simulink model "Seminar6_topic2"  (R2015b)
settings: Solver=VariableStepAuto  StartTime=0.0  StopTime=0.2  FixedStep=5e-8  MaxStep=1e-5  RelTol=1e-3  AbsTol=.01
libraries: powerlib x11, powerlib_meascontrol x1, simulink x1
settings Model: Creator=96547  LastModifiedBy=96547
settings DataIOCC: SaveFormat=Array  SignalLoggingSaveFormat=ModelDataLogs
settings OptimizationCC: InitFltsAndDblsToZero=on
settings DebuggingCC: SaveWithParameterizedLinksMsg=none  UnderspecifiedInitializationDetection=Classic  MergeDetectMultiDrivingBlocksExec=none  SignalResolutionControl=TryResolveAllWithWarning  SolverPrmCheckMsg=warning  MultiTaskDSMMsg=warning  MultiTaskCondExecSysMsg=none  FcnCallInpInsideContextMsg=EnableAllAsWarning  UnconnectedInputMsg=none  UnconnectedOutputMsg=none  UnconnectedLineMsg=none  AllowSymbolicDim=on
settings HardwareCC: ProdBitPerPointer=32  ProdLargestAtomicFloat=None  ProdIntDivRoundTo=Undefined  ProdEndianess=Unspecified  ProdWordSize=32  ProdHWDeviceType=32-bit Generic
settings SFSimCC: SimUseLocalCustomCode=on
settings RTWCC: RTWUseLocalCustomCode=on
settings GRTTargetCC: TargetFcnLib=ansi_tfl_tmw.mat  CombineOutputUpdateFcns=off  GRTInterface=on
settings ConfigComp: CovModelRefEnable=Off  CovExternalEMLEnable=on

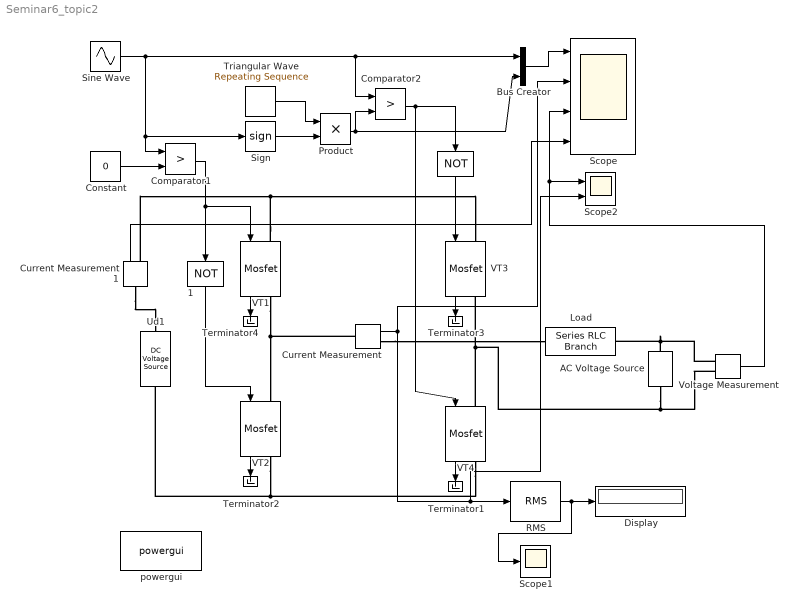
== system Seminar6_topic2 ==
  " " : Logic  Operator=NOT  AllPortsSameDT=off  OutDataTypeStr=boolean
  " 1" : Logic  Operator=NOT  AllPortsSameDT=off  OutDataTypeStr=boolean
  AC Voltage Source : powerlib/Electrical Sources/AC Voltage Source  Amplitude=220*sqrt(2)  Phase=0  Frequency=50  SampleTime=0  Measurements=None  BusType=swing  Pref=10e3  Qref=0  Qmin=-inf  Qmax=+inf
  Bus Creator : BusCreator  DialogController=Simulink.DDGSource_Bus  Inputs=2
  Comparator1 : RelationalOperator  Operator=>  OutDataTypeStr=boolean  ZeroCross=off
  Comparator2 : RelationalOperator  Operator=>  OutDataTypeStr=boolean  ZeroCross=off
  Constant : Constant  Value=0
  Current Measurement : powerlib/Measurements/Current Measurement  PhasorSimulation=off  OutputType=Complex  PSBequivalent=0
  Current Measurement1 : powerlib/Measurements/Current Measurement  PhasorSimulation=off  OutputType=Complex  PSBequivalent=0
  Display : Display
  Load : powerlib/Elements/Series RLC Branch  LConnTagsString=__new0  RConnTagsString=__new0  BranchType=RL  Resistance=0.1  Inductance=6e-3  SetiL0=off  InitialCurrent=0  Capacitance=inf  Setx0=off  InitialVoltage=0  Measurements=None
  Product : Product  RndMeth=Zero
  RMS : powerlib_meascontrol/Measurements/RMS  TrueRMS=on  Freq=50  RMSInit=0  Ts=0
  Scope : Scope  NumInputPorts=4
  Scope1 : Scope
  Scope2 : Scope  NumInputPorts=2
  Sign : Signum
  Sine Wave : Sin  Amplitude=0.590225  Frequency=100*pi  Phase=0.0814685  SampleTime=0
  Terminator{1..4} (4 alike) : Terminator
  Triangular Wave : simulink/Sources/Repeating Sequence  rep_seq_t=[0 2.5e-5 5e-5]  rep_seq_y=[1 0 1]
  Ud1 : powerlib/Electrical Sources/DC Voltage Source  Amplitude=630  Measurements=None
  VT{1..4} (4 alike) : powerlib/Power Electronics/Mosfet  Ron=0  Lon=1e-7  Rd=0  Vfd=0  IC=0  Rs=inf  Cs=inf  Measurements=on
  Voltage Measurement : powerlib/Measurements/Voltage Measurement  PhasorSimulation=off  OutputType=Complex  PSBequivalent=0
  powergui : powerlib/powergui  Priority=1  SimulationMode=Continuous  SampleTime=50e-6  frequency=60  Iterations=50  frequencyindice=50  Pbase=100e6  ErrMax=1e-4  UnitsV=kV  UnitsW=MW  buscounter=0  FunctionMessages=off  echomessages=off  EnableUseOfTLC=off  CurrentSourceSwitches=off  DisableSnubberDevices=off  DisableRonSwitches=off  DisableVfSwitches=off  DisplayEquations=off  AutomaticDiscreteSolvers=off  SolverType=Tustin/Backward Euler (TBE)  Interpol=off  ExternalGateDelay=off  methode=off  Ts=100  x0status=blocks  SPID=on  SwTol=0  HookPort=off  NonlinearTolerance=1e-4  nMaxIteration=100  ContinueOnMaxIteration=off  RestoreLinks=warning  ResistiveCurrentMeasurement=off  Frange=[0:2:500]  Ylog=off  Xlog=on  ShowGrid=off  save=off  variable=ZData  structure=0  ZoomFFT=off  StartTime=0.0  cycles=1  DisplayStyle=1  fundamental=60  FreqAxis=off  MaxFrequency=1000  frequencyindicesteady=1  RmsSteady=1  display=off
  wires:
  Comparator2/1 -> " "/1, VT4/1
  VT4/1 -> Terminator1/1
  VT2/1 -> Terminator2/1
  VT3/1 -> Terminator3/1
  Sine Wave/1 -> Sign/1, Comparator1/1, Bus Creator/1, Comparator2/1
  Bus Creator/1 -> Scope/1
  " "/1 -> VT3/1
  VT1/1 -> Terminator4/1
  Sign/1 -> Product/2
  " 1"/1 -> VT2/1
  Triangular Wave/1 -> Product/1
  Product/1 -> Comparator2/2, Bus Creator/2
  Comparator1/1 -> VT1/1, " 1"/1
  Constant/1 -> Comparator1/2
  Current Measurement/1 -> Scope/2, Scope2/2, RMS/1
  RMS/1 -> Scope1/1, Display/1
  Voltage Measurement/1 -> Scope/3, Scope2/1
  Current Measurement1/1 -> Scope/4
  connections:
  VT4/LConn1 -- AC Voltage Source/RConn1 -- Voltage Measurement/LConn2 -- VT3/RConn1
  VT1/RConn1 -- Current Measurement/LConn1 -- VT2/LConn1
  VT4/RConn1 -- Ud1/LConn1 -- VT2/RConn1
  VT1/LConn1 -- VT3/LConn1 -- Current Measurement1/RConn1
  AC Voltage Source/LConn1 -- Voltage Measurement/LConn1 -- Load/RConn1
  Current Measurement/RConn1 -- Load/LConn1
  Current Measurement1/LConn1 -- Ud1/RConn1
